simulink model "simulation"  (R2013b)
settings: Solver=ode45  StartTime=0.0  StopTime=2000  RelTol=1e-3
values from neighbouring files (symbols this model uses):
  delta = .5    (= 0.5)    [simulation_init.m]
  Fmax = 1000    [simulation_init.m]
  Fmin = -750    [simulation_init.m]
  J = I_z - N    (= 2752.5)    [simulation_init.m]
  k_r = .5    (= 0.5)    [simulation_init.m]
  k_u = .5    (= 0.5)    [simulation_init.m]
  k_xi = 1    [simulation_init.m]
  kl = diag([.05 .05 .001 100 100 100 100 100 100])    [simulation_init.m]
  kx = .3    (= 0.3)    [simulation_init.m]
  ky = .15    (= 0.15)    [simulation_init.m]
  kz = 1.5    [simulation_init.m]
  l = 1    [simulation_init.m]
  m_u = m - Xm_u    (= 4287.13636)    [simulation_init.m]
  m_uv = Xm_v - Xm_u    (= -28.713636)    [simulation_init.m]
  m_v = m - Xm_v    (= 4315.849996)    [simulation_init.m]
  n = 4    [simulation_init.m]
  noiseon = 1    [simulation_init.m]
  npsi = 0.00005    (= 5e-05)    [simulation_init.m]
  npsi_c = 0*.00005    (= 0)    [simulation_init.m]
  Nr = -110    [simulation_init.m]
  nr = 0.005    [simulation_init.m]
  Nrr = -555    [simulation_init.m]
  nsonar = .1    (= 0.1)    [simulation_init.m]
  nu = .05    (= 0.05)    [simulation_init.m]
  nv = 0.005    [simulation_init.m]
  nVc = 0*.005    (= 0)    [simulation_init.m]
  P01 = [20   20]    [simulation_init.m]
  P02 = [40   00]    [simulation_init.m]
  P03 = [20  -20]    [simulation_init.m]
  P04 = [150 40]    [simulation_init.m]
  psi01 = 0*pi/180    (= 0)    [simulation_init.m]
  psi02 = 0*pi/180    (= 0)    [simulation_init.m]
  psi03 = 0*pi/180    (= 0)    [simulation_init.m]
  psi_c = 45*pi/180    (= 0.785398163397)    [simulation_init.m]
  Q1 = diag([nu nv npsi nWvxy*ones(1,6)])    [simulation_init.m]
  Q2 = diag([nu nv npsi nWvxy*ones(1,6)])    [simulation_init.m]
  Q3 = diag([nu nv npsi nWvxy*ones(1,6)])    [simulation_init.m]
  Sigma01 = 15*eye(9)    [simulation_init.m]
  Sigma02 = Sigma01    [simulation_init.m]
  Sigma03 = Sigma01    [simulation_init.m]
  State_est01 = [P01+[sN(1),sN(2)] psi01 P02+[sN(3),sN(4)] P03+[sN(5),sN(6)]  P04 ]    [simulation_init.m]
  State_est02 = [P02+[sN(3),sN(4)] psi02 P01+[sN(1),sN(2)] P03+[sN(5),sN(6)]  P04 ]    [simulation_init.m]
  State_est03 = [P03+[sN(5),sN(6)] psi03 P01+[sN(1),sN(2)] P02+[sN(3),sN(5)]  P04 ]    [simulation_init.m]
  T_bc = 1    [simulation_init.m]
  T_est = .1    (= 0.1)    [simulation_init.m]
  Vc = .3    (= 0.3)    [simulation_init.m]
  Xu = -360    [simulation_init.m]
  Xuu = -805    [simulation_init.m]
  Yv = -420    [simulation_init.m]
  Yvv = -1930    [simulation_init.m]
undefined symbols (not defined in the file or in its folder): Pathdata
libraries: simulink x25
(part 2 of 2)

== system simulation/Vessel 3/Path Generator/Nominal Values Generator ==
  gam : Inport
  path params : Inport  Port=2
  Bus Selector : BusSelector  OutputSignals=gamWP,thetad,P0,v_L,Circle
  MATLAB Function : MATLAB Function  TreatAsAtomicUnit=on
  P_d : Outport
  dP_d : Outport  Port=2
  v_L : Outport  Port=3
  wires:
  path params/1 -> Bus Selector/1
  MATLAB Function/1(Pd) -> P_d/1
  MATLAB Function/2(dPd) -> dP_d/1
  gam/1 -> MATLAB Function/1(gam)
  Bus Selector/1 -> MATLAB Function/2(gamWP)  "<gamWP>"
  Bus Selector/2 -> MATLAB Function/3(thetad)  "<thetad>"
  Bus Selector/3 -> MATLAB Function/4(P0)  "<P0>"
  Bus Selector/4 -> v_L/1, MATLAB Function/5(v_L)  "<v_L>"
  Bus Selector/5 -> MATLAB Function/6(Radius)  "<Circle>"

== system simulation/Vessel 3/Path Generator/Read Pathdata ==
  gam : Inport
  pathdata : Inport  Port=2
  id : Inport  Port=3
  Bus Creator : BusCreator  Inputs=5
  Path1 : MATLAB Function  TreatAsAtomicUnit=on
  path params : Outport
  wires:
  gam/1 -> Path1/2(gam)
  Path1/3(P0) -> Bus Creator/3
  Path1/1(gamWP) -> Bus Creator/1
  Path1/2(thetad) -> Bus Creator/2
  Path1/4(v_L) -> Bus Creator/4
  Bus Creator/1 -> path params/1
  pathdata/1 -> Path1/1(pathdata)
  id/1 -> Path1/3(id)
  Path1/5(Circle) -> Bus Creator/5

== system simulation/Vessel 1/AUV/Dynamics/Propellers ==
  tau : Inport
  Demux1 : Demux  Outputs=2
  Fan forces : ToWorkspace  VariableName=F1  SampleTime=-1
  Gain : Gain  Gain=[.5 .5/l; .5 -.5/l]  Multiplication=Matrix(K*u)
  Saturation : Saturate  UpperLimit=Fmax  LowerLimit=Fmin
  Fs : Outport
  Fp : Outport  Port=2
  wires:
  Demux1/1 -> Fs/1
  tau/1 -> Gain/1
  Demux1/2 -> Fp/1
  Gain/1 -> Saturation/1
  Saturation/1 -> Demux1/1, Fan forces/1

== system simulation/Vessel 1/AUV/Kinematics/Water Current ==
  Sum : Sum  Inputs=++|
  Sum1 : Sum  Inputs=|++
  Vc : Constant  Value=Vc
  Vc noise : simulink/Sources/Band-Limited White Noise  Cov=nVc*5  Ts=5  seed=[23341]
  Water current : MATLAB Function  TreatAsAtomicUnit=on
  psi_c : Constant  Value=psi_c
  psi_c noise : simulink/Sources/Band-Limited White Noise  Cov=npsi_c*5  Ts=5  seed=[256]
  Vcxy : Outport
  wires:
  psi_c noise/1 -> Sum1/2
  Vc noise/1 -> Sum/1
  Water current/1(Vcxy) -> Vcxy/1
  Sum/1 -> Water current/1(Vc)
  Sum1/1 -> Water current/2(psi_c)
  Vc/1 -> Sum/2
  psi_c/1 -> Sum1/1

== system simulation/Vessel 2/AUV/Dynamics/Propellers ==
  tau : Inport
  Demux1 : Demux  Outputs=2
  Fan forces : ToWorkspace  VariableName=F2  SampleTime=-1
  Gain : Gain  Gain=[.5 .5/l; .5 -.5/l]  Multiplication=Matrix(K*u)
  Saturation : Saturate  UpperLimit=Fmax  LowerLimit=Fmin
  Fs : Outport
  Fp : Outport  Port=2
  wires:
  Saturation/1 -> Fan forces/1, Demux1/1
  Gain/1 -> Saturation/1
  Demux1/2 -> Fp/1
  tau/1 -> Gain/1
  Demux1/1 -> Fs/1

== system simulation/Vessel 2/AUV/Kinematics/Water Current ==
  Sum : Sum  Inputs=++|
  Sum1 : Sum  Inputs=|++
  Vc : Constant  Value=Vc
  Vc noise : simulink/Sources/Band-Limited White Noise  Cov=nVc*5  Ts=5  seed=9568
  Water current : MATLAB Function  TreatAsAtomicUnit=on
  psi_c : Constant  Value=psi_c
  psi_c noise : simulink/Sources/Band-Limited White Noise  Cov=npsi_c*5  Ts=5  seed=446
  Vcxy : Outport
  wires:
  psi_c/1 -> Sum1/1
  Vc/1 -> Sum/2
  Sum1/1 -> Water current/2(psi_c)
  Sum/1 -> Water current/1(Vc)
  Water current/1(Vcxy) -> Vcxy/1
  Vc noise/1 -> Sum/1
  psi_c noise/1 -> Sum1/2

== system simulation/Vessel 3/AUV/Dynamics/Propellers ==
  tau : Inport
  Demux1 : Demux  Outputs=2
  Fan forces : ToWorkspace  VariableName=F3  SampleTime=-1
  Gain : Gain  Gain=[.5 .5/l; .5 -.5/l]  Multiplication=Matrix(K*u)
  Saturation : Saturate  UpperLimit=Fmax  LowerLimit=Fmin
  Fs : Outport
  Fp : Outport  Port=2
  wires:
  Demux1/1 -> Fs/1
  tau/1 -> Gain/1
  Demux1/2 -> Fp/1
  Gain/1 -> Saturation/1
  Saturation/1 -> Demux1/1, Fan forces/1

== system simulation/Vessel 3/AUV/Kinematics/Water Current ==
  Sum : Sum  Inputs=++|
  Sum1 : Sum  Inputs=|++
  Vc : Constant  Value=Vc
  Vc noise : simulink/Sources/Band-Limited White Noise  Cov=nVc*5  Ts=5  seed=9864
  Water current : MATLAB Function  TreatAsAtomicUnit=on
  psi_c : Constant  Value=psi_c
  psi_c noise : simulink/Sources/Band-Limited White Noise  Cov=npsi_c*5  Ts=5  seed=2348
  Vcxy : Outport
  wires:
  psi_c noise/1 -> Sum1/2
  Vc noise/1 -> Sum/1
  Water current/1(Vcxy) -> Vcxy/1
  Sum/1 -> Water current/1(Vc)
  Sum1/1 -> Water current/2(psi_c)
  Vc/1 -> Sum/2
  psi_c/1 -> Sum1/1

== matlab function simulation/Vessel 1/AUV/Controller/Controller ==
  data: ud input; rd input; k_u parameter; k_r parameter; u input; tau output; v input; r input; m_u parameter; m_v parameter; m_uv parameter; J parameter; Xu parameter; Xuu parameter; Nr parameter; Nrr parameter
function tau = fcn(ud,rd,k_u,k_r,u,v,r,m_u,m_v,m_uv,J,Xu,Xuu,Nr,Nrr) 

d_u = -Xu - Xuu*abs(u);
d_r = -Nr - Nrr*abs(r);

tau_u = m_u*k_u*tanh(ud - u) + d_u*u - m_v*v*r;
tau_r = J*k_r*tanh(rd - r) + d_r*r - m_uv*u*v;

tau = [tau_u tau_r]';

== matlab function simulation/Vessel 1/AUV/Dynamics/Dynamics ==
  data: u input; dU output; v input; r input; Fs input; Fp input; m_u parameter; m_v parameter; m_uv parameter; J parameter; l parameter; Xu parameter; Xuu parameter; Yv parameter; Yvv parameter; Nr parameter; Nrr parameter
function dU = fcn(u,v,r,Fs,Fp,m_u,m_v,m_uv,J,l,Xu,Xuu,Yv,Yvv,Nr,Nrr) 

d_u = -Xu - Xuu*abs(u);
d_v = -Yv - Yvv*abs(v);
d_r = -Nr - Nrr*abs(r);

du = (m_v*v*r - d_u*u + Fs + Fp)/m_u;
dv = (-m_u*u*r - d_v*v)/m_v;
dr = (m_uv*u*v - d_r*r + l*(Fs - Fp))/J;

dU = [du dv dr]';

== matlab function simulation/Vessel 1/AUV/Kinematics/Kinematics ==
  data: Utot output; u input size=1; v input size=1; psi input size=1; dP output; Vc input size=2
function [Utot,dP]= fcn(u,v,psi,Vc)

R = [cos(psi) -sin(psi); sin(psi) cos(psi)];
dP = R*[u v]' + Vc;
Utot = sqrt(dP(1)^2 + dP(2)^2);

== matlab function simulation/Vessel 1/AUV/Kinematics/Water Current/Water current ==
  data: Vc input; Vcxy output; psi_c input
function Vcxy = fcn(Vc,psi_c)

Vcxy = Vc*[cos(psi_c); sin(psi_c)];

== matlab function simulation/Vessel 2/AUV/Controller/Controller ==
  data: ud input; rd input; k_u parameter; k_r parameter; u input; tau output; v input; r input; m_u parameter; m_v parameter; m_uv parameter; J parameter; Xu parameter; Xuu parameter; Nr parameter; Nrr parameter
function tau = fcn(ud,rd,k_u,k_r,u,v,r,m_u,m_v,m_uv,J,Xu,Xuu,Nr,Nrr) 

d_u = -Xu - Xuu*abs(u);
d_r = -Nr - Nrr*abs(r);

tau_u = m_u*k_u*tanh(ud - u) + d_u*u - m_v*v*r;
tau_r = J*k_r*tanh(rd - r) + d_r*r - m_uv*u*v;

tau = [tau_u tau_r]';

== matlab function simulation/Vessel 2/AUV/Dynamics/Dynamics ==
  data: u input; dU output; v input; r input; Fs input; Fp input; m_u parameter; m_v parameter; m_uv parameter; J parameter; l parameter; Xu parameter; Xuu parameter; Yv parameter; Yvv parameter; Nr parameter; Nrr parameter
function dU = fcn(u,v,r,Fs,Fp,m_u,m_v,m_uv,J,l,Xu,Xuu,Yv,Yvv,Nr,Nrr) 

d_u = -Xu - Xuu*abs(u);
d_v = -Yv - Yvv*abs(v);
d_r = -Nr - Nrr*abs(r);

du = (m_v*v*r - d_u*u + Fs + Fp)/m_u;
dv = (-m_u*u*r - d_v*v)/m_v;
dr = (m_uv*u*v - d_r*r + l*(Fs - Fp))/J;

dU = [du dv dr]';

== matlab function simulation/Vessel 2/AUV/Kinematics/Kinematics ==
  data: Utot output; u input size=1; v input size=1; psi input size=1; dP output; Vc input size=2
function [Utot,dP]= fcn(u,v,psi,Vc)

R = [cos(psi) -sin(psi); sin(psi) cos(psi)];
dP = R*[u v]' + Vc;
Utot = sqrt(dP(1)^2 + dP(2)^2);

== matlab function simulation/Vessel 2/AUV/Kinematics/Water Current/Water current ==
  data: Vc input; Vcxy output; psi_c input
function Vcxy = fcn(Vc,psi_c)

Vcxy = Vc*[cos(psi_c); sin(psi_c)];

== matlab function simulation/Vessel 2/Coordination Controller ==
  data: Gam_est input; v_tilde output; n parameter; k_xi parameter; i parameter
function v_tilde = fcn(Gam_est,n,k_xi,i)
assert(n<20);
D = diag((n-1)*ones(1,n));
A = ones(n) - eye(n); 
L_d = D\(D-A);
V_tilde = -k_xi * tanh(L_d*Gam_est);
v_tilde = V_tilde(i);

== matlab function simulation/Vessel 2/Coordination State Estimator/Update  ==
  data: Gam_predict input; gam_i input; Gam_est output; gam_j input; i parameter; j input
function Gam_est = fcn(Gam_predict,gam_i,gam_j,i,j)
%#codegen
Gam_est = Gam_predict;
Gam_est(i) = gam_i;
if gam_j ~= 0
    Gam_est(j) = gam_j;
end

== matlab function simulation/Vessel 2/Path Generator/Nominal Values Generator/MATLAB Function ==
  data: gam input; Pd output; gamWP input; dPd output; thetad input; P0 input; v_L input; Radius input
function [Pd,dPd] = fcn(gam, gamWP,thetad,P0,v_L,Radius)
%#codegen
if Radius ~= 0
    R0 = P0;
    R = Radius;
    alpha0 = thetad;
    dPd = [0;0];
    dPd(1) = -sin(alpha0 + (gam-gamWP)*v_L/R)*v_L;
    dPd(2) =  cos(alpha0 + (gam-gamWP)*v_L/R)*v_L;
    Pd = R0 + [cos(alpha0 + (gam-gamWP)*v_L/R)*R;...
                sin(alpha0 + (gam-gamWP)*v_L/R)*R];
else
    dPd = [0;0];
    dPd(1) = cos(thetad)*v_L;
    dPd(2) = sin(thetad)*v_L;
    Pd = P0 + dPd*(gam-gamWP);
end

== matlab function simulation/Vessel 2/Path Generator/Read Pathdata/Path1 ==
  data: pathdata input; gam input; gamWP output; thetad output; P0 output; v_L output; id input; Circle output
function [gamWP,thetad,P0,v_L,Circle]  =  fcn(pathdata,gam,id)

if      gam >=0 && gam < pathdata(1,2,id)
        pdataiStep = pathdata(:,1,id);
elseif  gam >=pathdata(1,2,id) && gam < pathdata(1,3,id)
        pdataiStep = pathdata(:,2,id);
elseif  gam >=pathdata(1,3,id) && gam < pathdata(1,4,id)
        pdataiStep = pathdata(:,3,id);
elseif  gam >=pathdata(1,4,id) && gam < pathdata(1,5,id)
        pdataiStep = pathdata(:,4,id);
elseif  gam >=pathdata(1,5,id) && gam < pathdata(1,6,id)
        pdataiStep = pathdata(:,5,id);
else
    pdataiStep = pathdata(:,6,id);
end

    gamWP   = pdataiStep(1);
    thetad     = pdataiStep(2); 
    P0      =  [pdataiStep(3);pdataiStep(4)]; 
    v_L    = pdataiStep(5);
    Circle    = pdataiStep(6);

== matlab function simulation/Vessel 2/Path-Following Controller/PF Control Law ==
  data: Vc input size=2; P input size=2; psi input size=1; kx parameter; ky parameter; kz parameter; Pd input size=2; dPd input size=2; Vd input size=1; delta parameter; Ud output size=2; e output size=2; dgam input size=1; ddgam output size=1
function [Ud,e,ddgam] = fcn(Vc,P,psi,kx,ky,kz,Pd,dPd,Vd,delta,dgam)


R = [cos(psi) -sin(psi); sin(psi) cos(psi)];
e = R'*(Pd - P);
d = [delta; 0];
z = dgam - Vd;

Ud = [1 0; 0 1/delta]*([kx 0; 0 ky]*tanh(e - d) - R'*Vc + Vd*R'*dPd);
ddgam = -kz*z - (e - d)'*R'*dPd;

== matlab function simulation/Vessel 2/State Estimator/State prediction ==
  data: Sigma_km1 input; State_km1 input; T_est parameter; Vc input; Q input; Psi input; Usens input; State_predict output; Sigma_predict output
function [State_predict,Sigma_predict] = fcn(Sigma_km1,State_km1,T_est,Vc,Q, Psi,Usens)
%#codegen
% Variables
u = Usens(1);
v = Usens(2);

% Linearization
F_km1 = [1 0 0 0 0 0 0 0 0;...
         0 1 0 0 0 0 0 0 0;...
         0 0 0 0 0 0 0 0 0;...
         0 0 0 1 0 0 0 0 0;...
         0 0 0 0 1 0 0 0 0;...
         0 0 0 0 0 1 0 0 0;...
         0 0 0 0 0 0 1 0 0;...
         0 0 0 0 0 0 0 1 0;...
         0 0 0 0 0 0 0 0 1];         
     
U_km1 = [cos(Psi)*T_est     -sin(Psi)*T_est     (-u*sin(Psi)-v*cos(Psi))*T_est zeros(1,6);...
         sin(Psi)*T_est     cos(Psi)*T_est      (u*cos(Psi)-v*sin(Psi))*T_est  zeros(1,6);...
         0                  0                    1                        zeros(1,6);...
         0                  0                    0                             T_est 0 0 0 0 0;...
         0                  0                    0                             0 T_est 0 0 0 0;...
         0                  0                    0                             0 0 T_est 0 0 0;...
         0                  0                    0                             0 0 0 T_est 0 0;...
         0                  0                    0                             0 0 0 0 T_est 0;...
         0                  0                    0                             0 0 0 0 0 T_est];

         
     
% State Dynamics
State_predict = F_km1*State_km1 +...
                [Vc(1)*T_est; Vc(2)*T_est; 0; zeros(6,1)] +...
                [(u*cos(Psi) - v*sin(Psi))*T_est; (u*sin(Psi) + v*cos(Psi))*T_est; Psi; zeros(6,1)];
            
% Covariance Dynamics
Sigma_predict = F_km1 * Sigma_km1 * F_km1' + U_km1*Q*U_km1';

== matlab function simulation/Vessel 2/State Estimator/State update ==
  data: Sigma output; state_predict input; Sigma_predict input; z input; state_est output; covl input; statel input; nsonar parameter; j input; i parameter; state_i output; cov_i output; kl parameter
function [Sigma,state_est, state_i, cov_i] = fcn(state_predict,Sigma_predict, z, covl, statel, nsonar, j, i, kl)
%#codegen

% No State update
state_est = state_predict;
% No Covariance update
Sigma = Sigma_predict;
% Internal mapping
if j == i
    l = 0;
elseif j>i
    l = j-1;
else
    l =j;
end
assert (l<=5);
if l>5 || l<1
    l = 1;
end
covll = zeros(4,1);

% if measurement and reference from other! boat available
if i~=j && z>20*nsonar

        % Instant Update
        covll = covl;
        Pl = reshape(covll,2,2);
        Sigma_predict(2*l+2:2*l+3,2*l+2:2*l+3) = Pl;
        
        
        
        xh   = state_predict(1);
        yh   = state_predict(2);
        xlh  = statel(1);
        ylh  = statel(2);
        state_predict(2*l+2) = xlh;
        state_predict(2*l+3) = ylh;

        % Linearization
        dxhat = xh - xlh;
        dyhat = yh - ylh;
        % Measurement Prediction
        rhat  = sqrt(dxhat^2 + dyhat^2);
        H = [dxhat/rhat dyhat/rhat 0 zeros(1,2*l-2) -dxhat/rhat -dyhat/rhat    zeros(1,4-(2*l-2))];
         
         % Measurement Covariance
         R = 100*nsonar;
    
         % Measurement covariance prediction
        S = H*Sigma_predict*H' + R;
        % Filter Gain
        K = kl*tanh(kl\Sigma_predict*H'/S);
        % Innovation
        lambda = z - rhat;
        % State update
        state_est = state_predict + K*lambda;
        % Covariance update
        Sigma = Sigma_predict - K*H*Sigma_predict;

end

state_i = state_est(1:2);
cov11 = Sigma(1:2,1:2);
cov_i = cov11(:);

== matlab function simulation/Vessel 3/AUV/Controller/Controller ==
  data: ud input; rd input; k_u parameter; k_r parameter; u input; tau output; v input; r input; m_u parameter; m_v parameter; m_uv parameter; J parameter; Xu parameter; Xuu parameter; Nr parameter; Nrr parameter
function tau = fcn(ud,rd,k_u,k_r,u,v,r,m_u,m_v,m_uv,J,Xu,Xuu,Nr,Nrr) 

d_u = -Xu - Xuu*abs(u);
d_r = -Nr - Nrr*abs(r);

tau_u = m_u*k_u*tanh(ud - u) + d_u*u - m_v*v*r;
tau_r = J*k_r*tanh(rd - r) + d_r*r - m_uv*u*v;

tau = [tau_u tau_r]';

== matlab function simulation/Vessel 1/Coordination Controller ==
  data: Gam_est input; v_tilde output; n parameter; k_xi parameter; i parameter
function v_tilde = fcn(Gam_est,n,k_xi,i)
assert(n<20);
D = diag((n-1)*ones(1,n));
A = ones(n) - eye(n); 
L_d = D\(D-A);
V_tilde = -k_xi * tanh(L_d*Gam_est);
v_tilde = V_tilde(i);

== matlab function simulation/Vessel 1/Coordination State Estimator/Update  ==
  data: Gam_predict input; gam_i input; Gam_est output; gam_j input; i parameter; j input
function Gam_est = fcn(Gam_predict,gam_i,gam_j,i,j)
%#codegen
Gam_est = Gam_predict;
Gam_est(i) = gam_i;
if gam_j ~= 0
    Gam_est(j) = gam_j;
end

== matlab function simulation/Vessel 3/AUV/Dynamics/Dynamics ==
  data: u input; dU output; v input; r input; Fs input; Fp input; m_u parameter; m_v parameter; m_uv parameter; J parameter; l parameter; Xu parameter; Xuu parameter; Yv parameter; Yvv parameter; Nr parameter; Nrr parameter
function dU = fcn(u,v,r,Fs,Fp,m_u,m_v,m_uv,J,l,Xu,Xuu,Yv,Yvv,Nr,Nrr) 

d_u = -Xu - Xuu*abs(u);
d_v = -Yv - Yvv*abs(v);
d_r = -Nr - Nrr*abs(r);

du = (m_v*v*r - d_u*u + Fs + Fp)/m_u;
dv = (-m_u*u*r - d_v*v)/m_v;
dr = (m_uv*u*v - d_r*r + l*(Fs - Fp))/J;

dU = [du dv dr]';

== matlab function simulation/Vessel 3/AUV/Kinematics/Kinematics ==
  data: Utot output; u input size=1; v input size=1; psi input size=1; dP output; Vc input size=2
function [Utot,dP]= fcn(u,v,psi,Vc)

R = [cos(psi) -sin(psi); sin(psi) cos(psi)];
dP = R*[u v]' + Vc;
Utot = sqrt(dP(1)^2 + dP(2)^2);

== matlab function simulation/Vessel 1/Path Generator/Nominal Values Generator/MATLAB Function ==
  data: gam input; Pd output; gamWP input; dPd output; thetad input; P0 input; v_L input; Radius input
function [Pd,dPd] = fcn(gam, gamWP,thetad,P0,v_L,Radius)
%#codegen
if Radius ~= 0
    R0 = P0;
    R = Radius;
    alpha0 = thetad;
    dPd = [0;0];
    dPd(1) = -sin(alpha0 + (gam-gamWP)*v_L/R)*v_L;
    dPd(2) =  cos(alpha0 + (gam-gamWP)*v_L/R)*v_L;
    Pd = R0 + [cos(alpha0 + (gam-gamWP)*v_L/R)*R;...
                sin(alpha0 + (gam-gamWP)*v_L/R)*R];
else
    dPd = [0;0];
    dPd(1) = cos(thetad)*v_L;
    dPd(2) = sin(thetad)*v_L;
    Pd = P0 + dPd*(gam-gamWP);
end

== matlab function simulation/Vessel 3/AUV/Kinematics/Water Current/Water current ==
  data: Vc input; Vcxy output; psi_c input
function Vcxy = fcn(Vc,psi_c)

Vcxy = Vc*[cos(psi_c); sin(psi_c)];

== matlab function simulation/Vessel 3/Coordination Controller ==
  data: Gam_est input; v_tilde output; n parameter; k_xi parameter; i parameter
function v_tilde = fcn(Gam_est,n,k_xi,i)
assert(n<20);
D = diag((n-1)*ones(1,n));
A = ones(n) - eye(n); 
L_d = D\(D-A);
V_tilde = -k_xi * tanh(L_d*Gam_est);
v_tilde = V_tilde(i);

== matlab function simulation/Vessel 1/Path Generator/Read Pathdata/Path1 ==
  data: pathdata input; gam input; gamWP output; thetad output; P0 output; v_L output; id input; Circle output
function [gamWP,thetad,P0,v_L,Circle]  =  fcn(pathdata,gam,id)

if      gam >=0 && gam < pathdata(1,2,id)
        pdataiStep = pathdata(:,1,id);
elseif  gam >=pathdata(1,2,id) && gam < pathdata(1,3,id)
        pdataiStep = pathdata(:,2,id);
elseif  gam >=pathdata(1,3,id) && gam < pathdata(1,4,id)
        pdataiStep = pathdata(:,3,id);
elseif  gam >=pathdata(1,4,id) && gam < pathdata(1,5,id)
        pdataiStep = pathdata(:,4,id);
elseif  gam >=pathdata(1,5,id) && gam < pathdata(1,6,id)
        pdataiStep = pathdata(:,5,id);
else
    pdataiStep = pathdata(:,6,id);
end

    gamWP   = pdataiStep(1);
    thetad     = pdataiStep(2); 
    P0      =  [pdataiStep(3);pdataiStep(4)]; 
    v_L    = pdataiStep(5);
    Circle    = pdataiStep(6);

== matlab function simulation/Vessel 3/Coordination State Estimator/Update  ==
  data: Gam_predict input; gam_i input; Gam_est output; gam_j input; i parameter; j input
function Gam_est = fcn(Gam_predict,gam_i,gam_j,i,j)
%#codegen
Gam_est = Gam_predict;
Gam_est(i) = gam_i;
if gam_j ~= 0
    Gam_est(j) = gam_j;
end

== matlab function simulation/Vessel 3/Path Generator/Nominal Values Generator/MATLAB Function ==
  data: gam input; Pd output; gamWP input; dPd output; thetad input; P0 input; v_L input; Radius input
function [Pd,dPd] = fcn(gam, gamWP,thetad,P0,v_L,Radius)
%#codegen
if Radius ~= 0
    R0 = P0;
    R = Radius;
    alpha0 = thetad;
    dPd = [0;0];
    dPd(1) = -sin(alpha0 + (gam-gamWP)*v_L/R)*v_L;
    dPd(2) =  cos(alpha0 + (gam-gamWP)*v_L/R)*v_L;
    Pd = R0 + [cos(alpha0 + (gam-gamWP)*v_L/R)*R;...
                sin(alpha0 + (gam-gamWP)*v_L/R)*R];
else
    dPd = [0;0];
    dPd(1) = cos(thetad)*v_L;
    dPd(2) = sin(thetad)*v_L;
    Pd = P0 + dPd*(gam-gamWP);
end

== matlab function simulation/Vessel 3/Path Generator/Read Pathdata/Path1 ==
  data: pathdata input; gam input; gamWP output; thetad output; P0 output; v_L output; id input; Circle output
function [gamWP,thetad,P0,v_L,Circle]  =  fcn(pathdata,gam,id)

if      gam >=0 && gam < pathdata(1,2,id)
        pdataiStep = pathdata(:,1,id);
elseif  gam >=pathdata(1,2,id) && gam < pathdata(1,3,id)
        pdataiStep = pathdata(:,2,id);
elseif  gam >=pathdata(1,3,id) && gam < pathdata(1,4,id)
        pdataiStep = pathdata(:,3,id);
elseif  gam >=pathdata(1,4,id) && gam < pathdata(1,5,id)
        pdataiStep = pathdata(:,4,id);
elseif  gam >=pathdata(1,5,id) && gam < pathdata(1,6,id)
        pdataiStep = pathdata(:,5,id);
else
    pdataiStep = pathdata(:,6,id);
end

    gamWP   = pdataiStep(1);
    thetad     = pdataiStep(2); 
    P0      =  [pdataiStep(3);pdataiStep(4)]; 
    v_L    = pdataiStep(5);
    Circle    = pdataiStep(6);

== matlab function simulation/Vessel 3/Path-Following Controller/PF Control Law ==
  data: Vc input size=2; P input size=2; psi input size=1; kx parameter; ky parameter; kz parameter; Pd input size=2; dPd input size=2; Vd input size=1; delta parameter; Ud output size=2; e output size=2; dgam input size=1; ddgam output size=1
function [Ud,e,ddgam] = fcn(Vc,P,psi,kx,ky,kz,Pd,dPd,Vd,delta,dgam)


R = [cos(psi) -sin(psi); sin(psi) cos(psi)];
e = R'*(Pd - P);
d = [delta; 0];
z = dgam - Vd;

Ud = [1 0; 0 1/delta]*([kx 0; 0 ky]*tanh(e - d) - R'*Vc + Vd*R'*dPd);
ddgam = -kz*z - (e - d)'*R'*dPd;

== matlab function simulation/Vessel 3/State Estimator/State prediction ==
  data: Sigma_km1 input; State_km1 input; T_est parameter; Vc input; Q input; Psi input; Usens input; State_predict output; Sigma_predict output
function [State_predict,Sigma_predict] = fcn(Sigma_km1,State_km1,T_est,Vc,Q, Psi,Usens)
%#codegen
% Variables
u = Usens(1);
v = Usens(2);

% Linearization
F_km1 = [1 0 0 0 0 0 0 0 0;...
         0 1 0 0 0 0 0 0 0;...
         0 0 0 0 0 0 0 0 0;...
         0 0 0 1 0 0 0 0 0;...
         0 0 0 0 1 0 0 0 0;...
         0 0 0 0 0 1 0 0 0;...
         0 0 0 0 0 0 1 0 0;...
         0 0 0 0 0 0 0 1 0;...
         0 0 0 0 0 0 0 0 1];         
     
U_km1 = [cos(Psi)*T_est     -sin(Psi)*T_est     (-u*sin(Psi)-v*cos(Psi))*T_est zeros(1,6);...
         sin(Psi)*T_est     cos(Psi)*T_est      (u*cos(Psi)-v*sin(Psi))*T_est  zeros(1,6);...
         0                  0                    1                        zeros(1,6);...
         0                  0                    0                             T_est 0 0 0 0 0;...
         0                  0                    0                             0 T_est 0 0 0 0;...
         0                  0                    0                             0 0 T_est 0 0 0;...
         0                  0                    0                             0 0 0 T_est 0 0;...
         0                  0                    0                             0 0 0 0 T_est 0;...
         0                  0                    0                             0 0 0 0 0 T_est];

         
     
% State Dynamics
State_predict = F_km1*State_km1 +...
                [Vc(1)*T_est; Vc(2)*T_est; 0; zeros(6,1)] +...
                [(u*cos(Psi) - v*sin(Psi))*T_est; (u*sin(Psi) + v*cos(Psi))*T_est; Psi; zeros(6,1)];
            
% Covariance Dynamics
Sigma_predict = F_km1 * Sigma_km1 * F_km1' + U_km1*Q*U_km1';

== matlab function simulation/Underwater Chanel/Calc Acoustic delays to range ==
  data: sonar input; dist output; map input; n parameter
function dist = fcn(sonar,map,n)
%#codegen
assert(n<20);
[sonarmax,i] = max(sonar); % sendingVessel
dist = zeros(4,1);
if sonarmax > 0
    for l = 1:n
        dist(l) = sqrt( (map(1,i)-map(1,l))^2 + (map(2,i)-map(2,l))^2);
    end
end

== matlab function simulation/Vessel 1/Path-Following Controller/PF Control Law ==
  data: Vc input size=2; P input size=2; psi input size=1; kx parameter; ky parameter; kz parameter; Pd input size=2; dPd input size=2; Vd input size=1; delta parameter; Ud output size=2; e output size=2; dgam input size=1; ddgam output size=1
function [Ud,e,ddgam] = fcn(Vc,P,psi,kx,ky,kz,Pd,dPd,Vd,delta,dgam)


R = [cos(psi) -sin(psi); sin(psi) cos(psi)];
e = R'*(Pd - P);
d = [delta; 0];
z = dgam - Vd;

Ud = [1 0; 0 1/delta]*([kx 0; 0 ky]*tanh(e - d) - R'*Vc + Vd*R'*dPd);
ddgam = -kz*z - (e - d)'*R'*dPd;

== matlab function simulation/Vessel 3/State Estimator/State update ==
  data: Sigma output; state_predict input; Sigma_predict input; z input; state_est output; covl input; statel input; nsonar parameter; j input; i parameter; state_i output; cov_i output; kl parameter
function [Sigma,state_est, state_i, cov_i] = fcn(state_predict,Sigma_predict, z, covl, statel, nsonar, j, i, kl)
%#codegen

% No State update
state_est = state_predict;
% No Covariance update
Sigma = Sigma_predict;
% Internal mapping
if j == i
    l = 0;
elseif j>i
    l = j-1;
else
    l =j;
end
assert (l<=5);
if l>5 || l<1
    l = 1;
end
covll = zeros(4,1);

% if measurement and reference from other! boat available
if i~=j && z>20*nsonar

        % Instant Update
        covll = covl;
        Pl = reshape(covll,2,2);
        Sigma_predict(2*l+2:2*l+3,2*l+2:2*l+3) = Pl;
        
        
        
        xh   = state_predict(1);
        yh   = state_predict(2);
        xlh  = statel(1);
        ylh  = statel(2);
        state_predict(2*l+2) = xlh;
        state_predict(2*l+3) = ylh;

        % Linearization
        dxhat = xh - xlh;
        dyhat = yh - ylh;
        % Measurement Prediction
        rhat  = sqrt(dxhat^2 + dyhat^2);
        H = [dxhat/rhat dyhat/rhat 0 zeros(1,2*l-2) -dxhat/rhat -dyhat/rhat    zeros(1,4-(2*l-2))];
         
         % Measurement Covariance
         R = 100*nsonar;
    
         % Measurement covariance prediction
        S = H*Sigma_predict*H' + R;
        % Filter Gain
        K = kl*tanh(kl\Sigma_predict*H'/S);
        % Innovation
        lambda = z - rhat;
        % State update
        state_est = state_predict + K*lambda;
        % Covariance update
        Sigma = Sigma_predict - K*H*Sigma_predict;

end

state_i = state_est(1:2);
cov11 = Sigma(1:2,1:2);
cov_i = cov11(:);

== matlab function simulation/Vessel 1/State Estimator/State prediction ==
  data: Sigma_km1 input; State_km1 input; T_est parameter; Vc input; Q input; Psi input; Usens input; State_predict output; Sigma_predict output
function [State_predict,Sigma_predict] = fcn(Sigma_km1,State_km1,T_est,Vc,Q, Psi,Usens)
%#codegen
% Variables
u = Usens(1);
v = Usens(2);

% Linearization
F_km1 = [1 0 0 0 0 0 0 0 0;...
         0 1 0 0 0 0 0 0 0;...
         0 0 0 0 0 0 0 0 0;...
         0 0 0 1 0 0 0 0 0;...
         0 0 0 0 1 0 0 0 0;...
         0 0 0 0 0 1 0 0 0;...
         0 0 0 0 0 0 1 0 0;...
         0 0 0 0 0 0 0 1 0;...
         0 0 0 0 0 0 0 0 1];         
     
U_km1 = [cos(Psi)*T_est     -sin(Psi)*T_est     (-u*sin(Psi)-v*cos(Psi))*T_est zeros(1,6);...
         sin(Psi)*T_est     cos(Psi)*T_est      (u*cos(Psi)-v*sin(Psi))*T_est  zeros(1,6);...
         0                  0                    1                        zeros(1,6);...
         0                  0                    0                             T_est 0 0 0 0 0;...
         0                  0                    0                             0 T_est 0 0 0 0;...
         0                  0                    0                             0 0 T_est 0 0 0;...
         0                  0                    0                             0 0 0 T_est 0 0;...
         0                  0                    0                             0 0 0 0 T_est 0;...
         0                  0                    0                             0 0 0 0 0 T_est];

         
     
% State Dynamics
State_predict = F_km1*State_km1 +...
                [Vc(1)*T_est; Vc(2)*T_est; 0; zeros(6,1)] +...
                [(u*cos(Psi) - v*sin(Psi))*T_est; (u*sin(Psi) + v*cos(Psi))*T_est; Psi; zeros(6,1)];
            
% Covariance Dynamics
Sigma_predict = F_km1 * Sigma_km1 * F_km1' + U_km1*Q*U_km1';

== matlab function simulation/Vessel 1/State Estimator/State update ==
  data: Sigma output; state_predict input; Sigma_predict input; z input; state_est output; covl input; statel input; nsonar parameter; j input; i parameter; state_i output; cov_i output; kl parameter
function [Sigma,state_est, state_i, cov_i] = fcn(state_predict,Sigma_predict, z, covl, statel, nsonar, j, i, kl)
%#codegen

% No State update
state_est = state_predict;
% No Covariance update
Sigma = Sigma_predict;
% Internal mapping
if j == i
    l = 0;
elseif j>i
    l = j-1;
else
    l =j;
end
assert (l<=5);
if l>5 || l<1
    l = 1;
end
covll = zeros(4,1);

% if measurement and reference from other! boat available
if i~=j && z>20*nsonar

        % Instant Update
        covll = covl;
        Pl = reshape(covll,2,2);
        Sigma_predict(2*l+2:2*l+3,2*l+2:2*l+3) = Pl;
        
        
        
        xh   = state_predict(1);
        yh   = state_predict(2);
        xlh  = statel(1);
        ylh  = statel(2);
        state_predict(2*l+2) = xlh;
        state_predict(2*l+3) = ylh;

        % Linearization
        dxhat = xh - xlh;
        dyhat = yh - ylh;
        % Measurement Prediction
        rhat  = sqrt(dxhat^2 + dyhat^2);
        H = [dxhat/rhat dyhat/rhat 0 zeros(1,2*l-2) -dxhat/rhat -dyhat/rhat    zeros(1,4-(2*l-2))];
         
         % Measurement Covariance
         R = 100*nsonar;
    
         % Measurement covariance prediction
        S = H*Sigma_predict*H' + R;
        % Filter Gain
        K = kl*tanh(kl\Sigma_predict*H'/S);
        % Innovation
        lambda = z - rhat;
        % State update
        state_est = state_predict + K*lambda;
        % Covariance update
        Sigma = Sigma_predict - K*H*Sigma_predict;

end

state_i = state_est(1:2);
cov11 = Sigma(1:2,1:2);
cov_i = cov11(:);
